simulink model "Hydraulic_Systemb_control101"  (R2023a)
settings: Solver=ode45  StartTime=0.0  StopTime=1000.0  RelTol=1e-3  EnableMultiTasking=on
undefined symbols (not defined in the file or in its folder): A1, a1, A2, a2, C1, C2, kp
settings Model: Creator=Mahmood  LastModifiedBy=Anthony Rossiter
settings SolverCC: AlgebraicLoopSolver=TrustRegion
settings DataIOCC: LimitDataPoints=on  SaveFormat=Array  SignalLoggingSaveFormat=ModelDataLogs  ReturnWorkspaceOutputs=off
settings OptimizationCC: BooleanDataType=off
settings DebuggingCC: SaveWithParameterizedLinksMsg=none  UnderspecifiedInitializationDetection=Classic  MergeDetectMultiDrivingBlocksExec=none  SignalResolutionControl=TryResolveAllWithWarning  MultiTaskDSMMsg=warning  MultiTaskCondExecSysMsg=none  UnconnectedInputMsg=warning  UnconnectedOutputMsg=warning  UnconnectedLineMsg=warning
settings HardwareCC: TargetUnknown=on
settings ModelReferenceCC: EnableRefExpFcnMdlSchedulingChecks=on  PropagateSignalLabelsOutOfModel=off
settings RTWCC: DLArmComputeVersion=19.05
settings GRTTargetCC: CombineOutputUpdateFcns=off  GRTInterface=on
settings ConfigComp: CovMetricSettings=dw

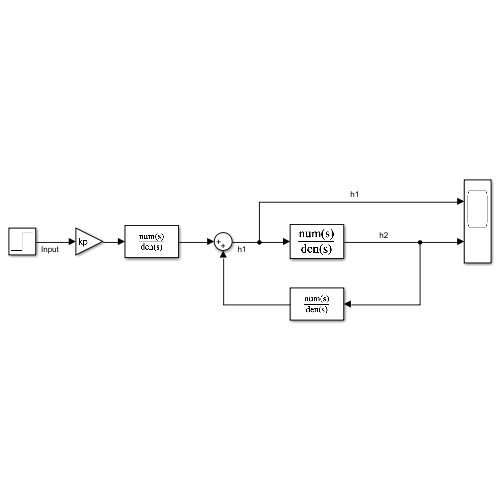
[thumbnail: Simulink's stored preview of the top-level diagram]
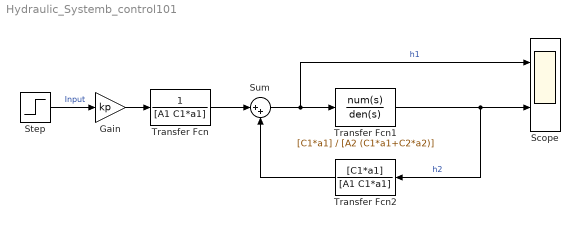
== system Hydraulic_Systemb_control101 ==
  Gain : Gain  Gain=kp  SaturateOnIntegerOverflow=on
  Scope : Scope  NumInputPorts=2
  Step : Step  After=3  SampleTime=0
  Sum : Sum  Inputs=|++  SaturateOnIntegerOverflow=on
  Transfer Fcn : TransferFcn  Denominator=[A1 C1*a1]
  Transfer Fcn1 : TransferFcn  Numerator=[C1*a1]  Denominator=[A2 (C1*a1+C2*a2)]
  Transfer Fcn2 : TransferFcn  Numerator=[C1*a1]  Denominator=[A1 C1*a1]
  wires:
  Step/1 -> Gain/1  "Input"
  Gain/1 -> Transfer Fcn/1
  Transfer Fcn/1 -> Sum/1
  Transfer Fcn1/1 -> Transfer Fcn2/1, Scope/2  "h2"
  Sum/1 -> Transfer Fcn1/1, Scope/1  "h1"
  Transfer Fcn2/1 -> Sum/2
